simulink subsystem "Piero_ControladoZ_memoria"  (R2023b)
settings: Solver=VariableStepAuto  StartTime=0.0  StopTime=10.0  RelTol=1e-3
settings Model: Creator=marqu  LastModifiedBy=marqu

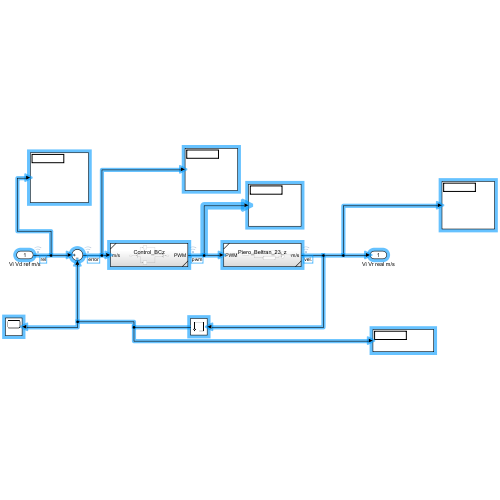
[thumbnail: Simulink's stored preview of the top-level diagram]
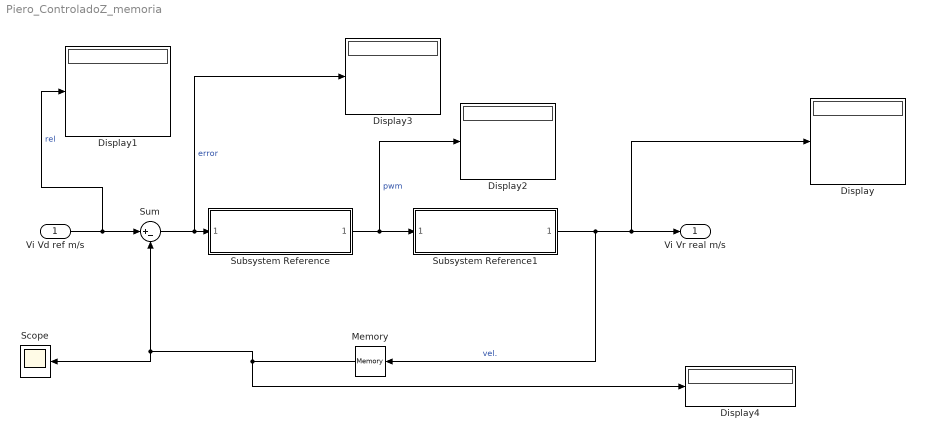
== system Piero_ControladoZ_memoria ==
  Vi Vd ref m/s : Inport
  Display{,1..4} (5 alike) : Display
  Memory : Memory
  Scope : Scope
  Subsystem Reference : Subsystem  ReferencedSubsystem=Control_BCz
  Subsystem Reference1 : Subsystem  ReferencedSubsystem=Piero_Beltran_23_z
  Sum : Sum  Inputs=|+-
  Vi Vr real m/s : Outport
  wires:
  Memory/1 -> Sum/2, Scope/1, Display4/1
  Subsystem Reference1/1 -> Memory/1, Display/1, Vi Vr real m/s/1  "vel."
  Sum/1 -> Display3/1, Subsystem Reference/1  "error"
  Vi Vd ref m/s/1 -> Display1/1, Sum/1  "rel"
  Subsystem Reference/1 -> Display2/1, Subsystem Reference1/1  "pwm"
